simulink model "phaser_simulink"  (R2023b)
settings: Solver=VariableStepAuto  StartTime=0.0  StopTime=10.0  RelTol=1e-3
libraries: dsparch4 x10, dspsnks4 x1, dspvision x1
settings Model: Creator=thv0  LastModifiedBy=thv0

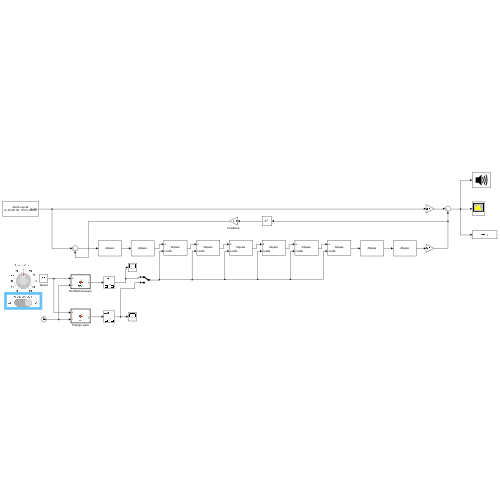
[thumbnail: Simulink's stored preview of the top-level diagram]
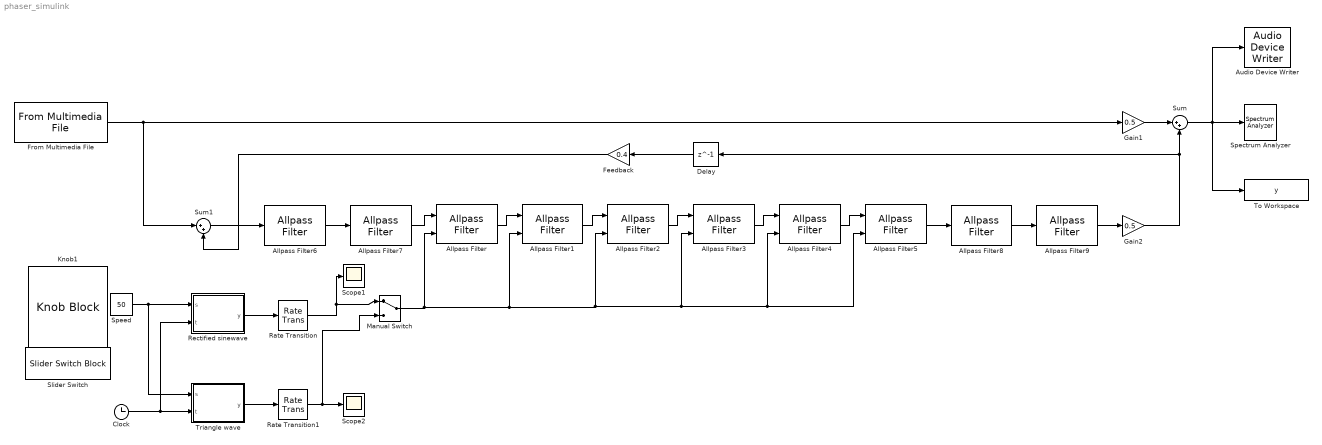
== system phaser_simulink ==
  Allpass Filter{,1..5} (6 alike) : dsparch4/Allpass Filter  Structure=Minimum multiplier  AllpassCoefficientsPort=on  AllpassCoefficients=[ -2^(-1/2), 1/2 ]  LatticeCoefficientsPort=off  LatticeCoefficients=[ -2^(1/2)/3, 1/2 ]  WDFCoefficients=[ 1/2, -2^(1/2)/3 ]  TrailingFirstOrderSection=off  SimulateUsing=Code generation
  Allpass Filter6 : dsparch4/Allpass Filter  Structure=Minimum multiplier  AllpassCoefficientsPort=off  AllpassCoefficients=[-0.89 ]  LatticeCoefficientsPort=off  LatticeCoefficients=[ -2^(1/2)/3, 1/2 ]  WDFCoefficients=[ 1/2, -2^(1/2)/3 ]  TrailingFirstOrderSection=off  SimulateUsing=Code generation
  Allpass Filter7 : dsparch4/Allpass Filter  Structure=Minimum multiplier  AllpassCoefficientsPort=off  AllpassCoefficients=[-0.89]  LatticeCoefficientsPort=off  LatticeCoefficients=[ -2^(1/2)/3, 1/2 ]  WDFCoefficients=[ 1/2, -2^(1/2)/3 ]  TrailingFirstOrderSection=off  SimulateUsing=Code generation
  Allpass Filter8 : dsparch4/Allpass Filter  Structure=Minimum multiplier  AllpassCoefficientsPort=off  AllpassCoefficients=[-0.89 ]  LatticeCoefficientsPort=off  LatticeCoefficients=[ -2^(1/2)/3, 1/2 ]  WDFCoefficients=[ 1/2, -2^(1/2)/3 ]  TrailingFirstOrderSection=off  SimulateUsing=Code generation
  Allpass Filter9 : dsparch4/Allpass Filter  Structure=Minimum multiplier  AllpassCoefficientsPort=off  AllpassCoefficients=[-0.89 ]  LatticeCoefficientsPort=off  LatticeCoefficients=[ -2^(1/2)/3, 1/2 ]  WDFCoefficients=[ 1/2, -2^(1/2)/3 ]  TrailingFirstOrderSection=off  SimulateUsing=Code generation
  Audio Device Writer : dspsnks4/Audio Device Writer  Driver=DirectSound  Device=OUT 1-2 (BEHRINGER UMC 202HD 192k)  InheritSampleRate=on  SampleRate=44100  BitDepth=16-bit integer  BufferSize=4096  NumBuffers=10  DefaultOutputChannelMapping=on  OutputChannelMapping=1:2  OutputNumUnderrunSamples=off  DriverIdx=1  DeviceWarnFlag=''
  Clock : Clock
  Delay : Delay  DelayLength=1  InitialCondition=0
  Feedback : Gain  Gain=0.4
  From Multimedia File : dspvision/From Multimedia File  inputFilename=D:\phaser\drumLoop.aif  readRange=[1 Inf]  loop=on  numPlays=inf  outputStreams=Audio only  videoDataType=single  audioDataType=double  inheritSampleTime=on  userDefinedSampleTime=1/30  noAudioOutput=off  isIntensityVideo=off  fourcc=RGB  colorVideoFormat=Separate color signals  outputEOF=off  dataOrg=Column-major  audioFrameSize=1024  computeAudioFrameSize=off  outSamplingMode=Sample based
      settings: LibrarySourceBlock=audiosources/From Multimedia File
  Gain1 : Gain  Gain=0.5
  Gain2 : Gain  Gain=0.5
  Knob1 : KnobBlock
  Manual Switch : ManualSwitch
  Rate Transition : RateTransition
  Rate Transition1 : RateTransition
  Rectified sinewave : MATLAB Function  TreatAsAtomicUnit=on
  Scope1 : Scope
  Scope2 : Scope
  Slider Switch : SliderSwitchBlock
      settings: Values={{'Off', 'On'}, [0 0.4]}
  Spectrum Analyzer : SpectrumAnalyzer  WindowPosition=[877.000000,775.000000,800.000000,445.000000,]  Visible=on  ScopeFrameLocation=window  SampleRateSource=Property  SampleRate=44.1e3  PlotAsTwoSidedSpectrum=off  FrequencyScale=Log  FrequencySpan=Start and stop frequencies  StartFrequency=20  StopFrequency=20e3  YLimits=[-81.94518552,3.92887182]
  Speed : Constant  Value=50
  Sum : Sum  Inputs=|++
  Sum1 : Sum  Inputs=|++
  To Workspace : ToWorkspace  VariableName=y  SaveFormat=Timeseries  SampleTime=-1
  Triangle wave : MATLAB Function  TreatAsAtomicUnit=on
  wires:
  Allpass Filter6/1 -> Allpass Filter7/1
  Allpass Filter7/1 -> Allpass Filter/1
  Allpass Filter/1 -> Allpass Filter1/1
  Allpass Filter1/1 -> Allpass Filter2/1
  Allpass Filter2/1 -> Allpass Filter3/1
  Allpass Filter3/1 -> Allpass Filter4/1
  Allpass Filter4/1 -> Allpass Filter5/1
  Allpass Filter5/1 -> Allpass Filter8/1
  Allpass Filter8/1 -> Allpass Filter9/1
  Sum/1 -> To Workspace/1, Spectrum Analyzer/1, Audio Device Writer/1
  Allpass Filter9/1 -> Gain2/1
  Rate Transition/1 -> Manual Switch/1, Scope1/1
  Manual Switch/1 -> Allpass Filter5/2, Allpass Filter4/2, Allpass Filter3/2, Allpass Filter2/2, Allpass Filter1/2, Allpass Filter/2
  Rate Transition1/1 -> Manual Switch/2, Scope2/1
  Speed/1 -> Triangle wave/1(s), Rectified sinewave/1(s)
  Rectified sinewave/1(y) -> Rate Transition/1
  Triangle wave/1(y) -> Rate Transition1/1
  Clock/1 -> Rectified sinewave/2(t), Triangle wave/2(t)
  Gain2/1 -> Delay/1, Sum/2
  Gain1/1 -> Sum/1
  Sum1/1 -> Allpass Filter6/1
  From Multimedia File/1 -> Sum1/1, Gain1/1
  Delay/1 -> Feedback/1
  Feedback/1 -> Sum1/2

== matlab function phaser_simulink/Rectified sinewave ==
  data: s input; y output; t input
function y = sine(s, t) % modulating wave gen
    f = 0.069 * exp(0.04*s);
    y = abs(sin(2*pi*f*t/2))*(1.26) - 0.49; % full wave rectified [-0.49, 0.77]

== matlab function phaser_simulink/Triangle wave ==
  data: s input; y output; t input
function y = tria(s, t) % modulating wave gen
    f = 0.069 * exp(0.04*s);
    y = sawtooth(2*pi*f*t, 0.5)*(0.225) - 0.615; % triangle wave [-0.84, -0.39]
